simulink model "MotorControl_Bldc"  (R2022a)
settings: Solver=ode4  StartTime=0.0  StopTime=1  FixedStep=Ts/cnt_pTs  RelTol=1e-3
values from neighbouring files (symbols this model uses):
  cnt_pTs = 1000    [motorpara.m]
  Fc = 1/Ts    (= 10000)    [motorpara.m]
  Ki_id = Rs*Fc    (= 4500)    [motorpara.m]
  Ki_iq = Rs*Fc    (= 4500)    [motorpara.m]
  Ki_v = 0.93    [motorpara.m]
  Kp_id = Ls*Fc    (= 4.2)    [motorpara.m]
  Kp_iq = Ls*Fc    (= 4.2)    [motorpara.m]
  Kp_v = 0.05    [motorpara.m]
  Ls = 0.00042    [motorpara.m]
  P = 2    [motorpara.m]
  Rs = 0.45    [motorpara.m]
  SMO_Kslide = 10    [motorpara.m]
  Ts = 1/10000    (= 0.0001)    [motorpara.m]
  V = 12    [motorpara.m]
undefined symbols (not defined in the file or in its folder): DiscIntNeverNeededParam, sigbuilder_block
libraries: nesl_utility x83, fl_lib x67, ee_lib x49, simulink x13, slpidlib x3, mcbplantlib x2, autolibpmsmexterior x1
(part 1 of 4)
settings Model: Creator=gcx  LastModifiedBy=gcx
settings OptimizationCC: DefaultParameterBehavior=Inlined  UseDivisionForNetSlopeComputation=on  GainParamInheritBuiltInType=on  UseFloatMulNetSlope=on  InlineInvariantSignals=on  PassReuseOutputArgsAs=Individual arguments  ZeroExternalMemoryAtStartup=off  ZeroInternalMemoryAtStartup=off  NoFixptDivByZeroProtection=on  EfficientFloat2IntCast=on  LifeSpan=1  OptimizeBlockOrder=speed  DifferentSizesBufferReuse=on  EfficientTunableParamExpr=on
settings DebuggingCC: ParameterTunabilityLossMsg=error
settings HardwareCC: ProdBitPerInt=16  ProdBitPerPointer=16  ProdBitPerSizeT=16  ProdBitPerPtrDiffT=16  ProdLargestAtomicFloat=None  ProdWordSize=16  ProdLongLongMode=on  ProdHWDeviceType=STMicroelectronics->ST10/Super10
settings SFSimCC: MATLABDynamicMemAlloc=off
settings RTWCC: SystemTargetFile=ert.tlc  GenCodeOnly=on  PackageGeneratedCodeAndArtifacts=on  TemplateMakefile=ert_default_tmf
settings CodeAppCC: ForceParamTrailComments=on  IgnoreCustomStorageClasses=off  OperatorAnnotations=on  SimulinkDataObjDesc=on  SFDataObjDesc=on  CustomSymbolStrGlobalVar=rt$N$M  CustomSymbolStrType=$N$M  CustomSymbolStrFcn=$N$M$F  CustomSymbolStrMacro=$N$M  InsertBlockDesc=on
settings ERTTargetCC: TargetLangStandard=C99 (ISO)  GenerateSampleERTMain=on  IncludeMdlTerminateFcn=off  CombineSignalStateStructs=on  CodeInterfacePackaging=Reusable function  SupportComplex=off  SupportNonInlinedSFcns=on  InlinedParameterPlacement=NonHierarchical  ERTCustomFileTemplate=example_file_process.tlc  ERTFilePackagingFormat=CompactWithDataFile

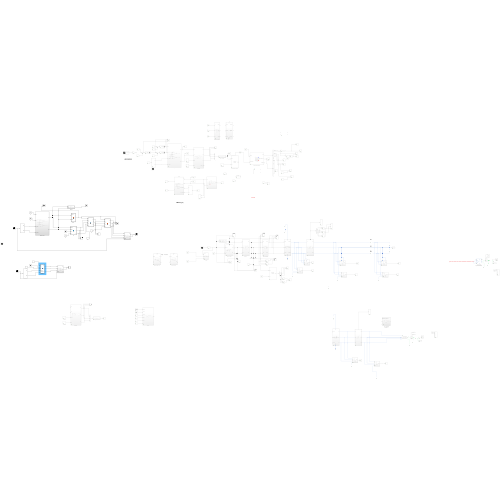
[thumbnail: Simulink's stored preview of the top-level diagram]
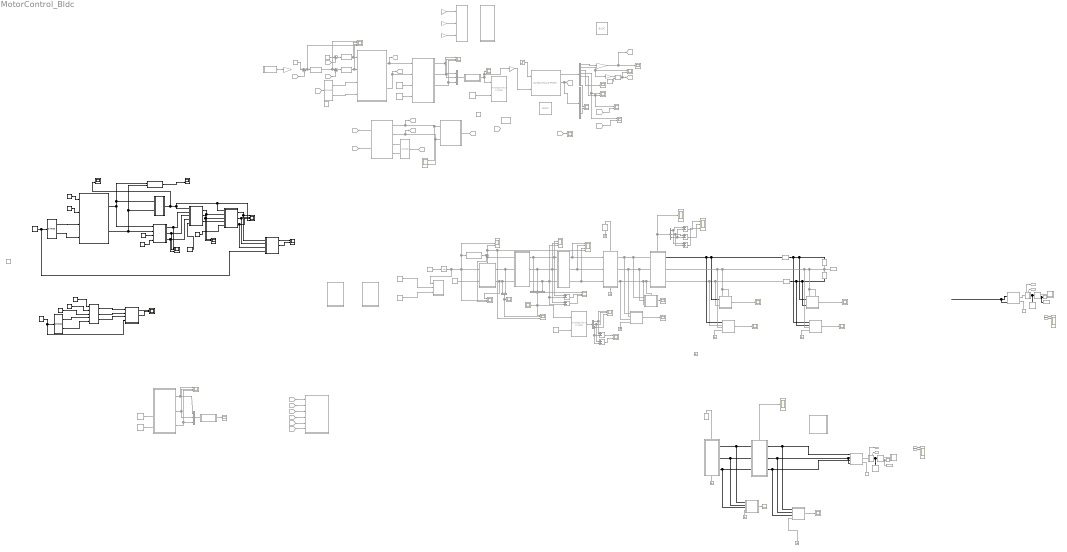
== system MotorControl_Bldc ==
  note: A
  note: 有Bug，可以用来还原
  note: Park变换
  note: 速度测量
  note: ）
  note: C
  note: B
  2Phase_D1D1 : Subsystem  Commented=on
      settings: PortSchema="{\"entries\":[{\"content\":{\"sides\":[{\"content\":{\"connectorIds\":[\"In1\",\"In2\"]},\"type\":\"ConnectorPlacement.EquallySpacedRectSide\",\"uuid\":\"91e4105a-9e8c-434e-97cb-db4fedd585cb\"},{\"content\":{\"connectorIds\":[\"Out1\",\"Out2\"],\"side\":\"RIGHT\"},\"type\":\"ConnectorPlacement.EquallySpacedRectSide\",\"uuid\":\"7c5735c0-a428-475d-8251-3447de6cb9b4\"},{\"content\":{\"connectorIds\":[\"In3\"],\"side\":\"TOP\"},\"type\":\"ConnectorPlacement.EquallySpacedRectSide\",\"uuid\":\"865a6bbc-fe0c-46ed-bd30-e6e1f24b581f\"}]},\"type\":\"ConnectorPlacement.EquallySpacedConnector\",\"uuid\":\"82a7eed4-0b98-4350-8284-359f4eec5efe\"}],\"packageUris\":[\"http://schema.mathworks.com/mf0/Connector/R2020b\"],\"version\":\"1.0\"}"
  2Phase_D1D1_org : Subsystem  Commented=on
      settings: PortSchema="{\"entries\":[{\"content\":{\"sides\":[{\"content\":{\"connectorIds\":[\"In1\",\"In2\"]},\"type\":\"ConnectorPlacement.EquallySpacedRectSide\",\"uuid\":\"91e4105a-9e8c-434e-97cb-db4fedd585cb\"},{\"content\":{\"connectorIds\":[\"Out1\",\"Out2\"],\"side\":\"RIGHT\"},\"type\":\"ConnectorPlacement.EquallySpacedRectSide\",\"uuid\":\"7c5735c0-a428-475d-8251-3447de6cb9b4\"},{\"content\":{\"connectorIds\":[\"In3\"],\"side\":\"TOP\"},\"type\":\"ConnectorPlacement.EquallySpacedRectSide\",\"uuid\":\"865a6bbc-fe0c-46ed-bd30-e6e1f24b581f\"}]},\"type\":\"ConnectorPlacement.EquallySpacedConnector\",\"uuid\":\"82a7eed4-0b98-4350-8284-359f4eec5efe\"}],\"packageUris\":[\"http://schema.mathworks.com/mf0/Connector/R2020b\"],\"version\":\"1.0\"}"
  2Phase_D1D2 : Subsystem  Commented=on
      settings: PortSchema="{\"entries\":[{\"content\":{\"sides\":[{\"content\":{\"connectorIds\":[\"In1\",\"In2\"]},\"type\":\"ConnectorPlacement.EquallySpacedRectSide\",\"uuid\":\"91e4105a-9e8c-434e-97cb-db4fedd585cb\"},{\"content\":{\"connectorIds\":[\"Out1\",\"Out2\"],\"side\":\"RIGHT\"},\"type\":\"ConnectorPlacement.EquallySpacedRectSide\",\"uuid\":\"7c5735c0-a428-475d-8251-3447de6cb9b4\"},{\"content\":{\"connectorIds\":[\"In3\"],\"side\":\"TOP\"},\"type\":\"ConnectorPlacement.EquallySpacedRectSide\",\"uuid\":\"865a6bbc-fe0c-46ed-bd30-e6e1f24b581f\"}]},\"type\":\"ConnectorPlacement.EquallySpacedConnector\",\"uuid\":\"82a7eed4-0b98-4350-8284-359f4eec5efe\"}],\"packageUris\":[\"http://schema.mathworks.com/mf0/Connector/R2020b\"],\"version\":\"1.0\"}"
  2Phase_T : Subsystem  Commented=on
  Add{2..5} (4 alike) : Sum  Commented=on  Inputs=+-
  Add6 : Sum  Commented=on
  Average-Value Inverter : mcbplantlib/Average-Value Inverter  Commented=on
  Average-Value Inverter1 : mcbplantlib/Average-Value Inverter  Commented=on
  BLDC : ee_lib/Electromechanical/Permanent Magnet/BLDC  Commented=on  port_option=ee.enum.threePhasePort.composite  winding_type=ee.enum.statorconnection.delta  rotor_param=ee.enum.pmsm.backemf.trapezoidflux  pm_flux_linkage=0.03 Wb  theta_constant=pi / 12 rad  emf_max=9.6 V  w_meas=600 rpm  DphiDtheta_tab=[0, -.1528, -.1528, .1528, .1528, 0] Wb/rad  back_emf_tab=[0, -9.6, -9.6, 9.6, 9.6, 0] V  rotor_angle_tab=[0, 7.5, 22.5, 37.5, 52.5, 60] deg  nPolePairs=6  axes_param=ee.enum.rotorangle.daxis  stator_param=ee.enum.statorparam.LdLqL0  machine_param=ee.enum.dqparameterization.constant  Ld=0.00022 H  Lq=0.00022 H  idVec=[-200, 0, 200] A  iqVec=[-200, 0, 200] A  LdMatrix=0.00022 * ones(3, 3) H  LqMatrix=0.00022 * ones(3, 3) H  L0=0.00016 H  Ls=0.0002 H  Lm=0 H  Ms=0.00002 H  Rs=0.013 Ohm  zero_sequence=ee.enum.park.zerosequence.include  loss_param=ee.enum.ironloss.none  losses_oc=[0, 0, 0] W  losses_sc=[0, 0, 0] W  f_losses=60 Hz  Isc_losses=95 A  J=0.01 kg*m^2  lam=0 N*m*s/rad  i_d_specify=off  i_d_priority=None  i_d=0 A  i_d_nominal_specify=off  i_d_nominal_unit=A  i_d_nominal_value=1  i_q_specify=off  i_q_priority=None  i_q=0 A  i_q_nominal_specify=off  i_q_nominal_unit=A  i_q_nominal_value=1  torque_specify=off  torque_priority=None  torque=0 N*m  torque_nominal_specify=off  torque_nominal_unit=N*m  torque_nominal_value=1  angular_velocity_specify=off  angular_velocity_priority=High  angular_velocity=0 rpm  angular_velocity_nominal_specify=off  angular_velocity_nominal_unit=rpm  angular_velocity_nominal_value=1  angular_position_specify=off  angular_position_priority=High  angular_position=0 deg  angular_position_nominal_specify=off  angular_position_nominal_unit=deg  angular_position_nominal_value=1  alpha=3.93e-3 1/K  alpha_flux=-0.001 1/K  Tmeas=298.15 K  stator_thermal_mass=100 J/K  rotor_thermal_mass=200 J/K  Rm_percent_rotor=90  Rd_percent_rotor=30  temperatureA_specify=off  temperatureA_priority=High  temperatureA=25 degC  temperatureA_nominal_specify=off  temperatureA_nominal_unit=degC  temperatureA_nominal_value=1  temperatureB_specify=off  temperatureB_priority=High  temperatureB=25 degC  temperatureB_nominal_specify=off  temperatureB_nominal_unit=degC  temperatureB_nominal_value=1  temperatureC_specify=off  temperatureC_priority=High  temperatureC=25 degC  temperatureC_nominal_specify=off  temperatureC_nominal_unit=degC  temperatureC_nominal_value=1  temperatureR_specify=off  temperatureR_priority=High  temperatureR=25 degC  temperatureR_nominal_specify=off  temperatureR_nominal_unit=degC  temperatureR_nominal_value=1
      settings: SourceProductBaseCode=PS  InternalSimscapePortConfiguration="{\"Bottom\":[],\"Left\":[{\"id\":\"N\",\"label\":\"~\",\"type\":\"foundation.electrical.three_phase\"},{\"id\":\"HR\",\"label\":\"HR\",\"type\":\"foundation.thermal.thermal\"}],\"Right\":[{\"id\":\"R\",\"label\":\"R\",\"type\":\"foundation.mechanical.rotational.rotational\"},{\"id\":\"C\",\"label\":\"C\",\"type\":\"foundation.mechanical.rotational.rotational\"},{\"id\":\"HA\",\"label\":\"HA\",\"type\":\"foundation.thermal.thermal\"},{\"id\":\"HB\",\"label\":\"HB\",\"type\":\"foundation.thermal.thermal\"},{\"id\":\"HC\",\"label\":\"HC\",\"type\":\"foundation.thermal.thermal\"}],\"Top\":[]}"
  BLDC1 : ee_lib/Electromechanical/Permanent Magnet/BLDC  Commented=on  port_option=ee.enum.threePhasePort.composite  winding_type=ee.enum.statorconnection.wye  rotor_param=ee.enum.pmsm.backemf.trapezoidflux  pm_flux_linkage=0.03 Wb  theta_constant=pi / 12 rad  emf_max=9.6 V  w_meas=600 rpm  DphiDtheta_tab=[0, -.1528, -.1528, .1528, .1528, 0] Wb/rad  back_emf_tab=[0, -9.6, -9.6, 9.6, 9.6, 0] V  rotor_angle_tab=[0, 7.5, 22.5, 37.5, 52.5, 60] deg  nPolePairs=6  axes_param=ee.enum.rotorangle.daxis  stator_param=ee.enum.statorparam.LdLqL0  machine_param=ee.enum.dqparameterization.constant  Ld=0.00022 H  Lq=0.00022 H  idVec=[-200, 0, 200] A  iqVec=[-200, 0, 200] A  LdMatrix=0.00022 * ones(3, 3) H  LqMatrix=0.00022 * ones(3, 3) H  L0=0.00016 H  Ls=0.0002 H  Lm=0 H  Ms=0.00002 H  Rs=0.013 Ohm  zero_sequence=ee.enum.park.zerosequence.include  loss_param=ee.enum.ironloss.none  losses_oc=[0, 0, 0] W  losses_sc=[0, 0, 0] W  f_losses=60 Hz  Isc_losses=95 A  J=0.01 kg*m^2  lam=0 N*m*s/rad  i_d_specify=off  i_d_priority=None  i_d=0 A  i_d_nominal_specify=off  i_d_nominal_unit=A  i_d_nominal_value=1  i_q_specify=off  i_q_priority=None  i_q=0 A  i_q_nominal_specify=off  i_q_nominal_unit=A  i_q_nominal_value=1  torque_specify=off  torque_priority=None  torque=0 N*m  torque_nominal_specify=off  torque_nominal_unit=N*m  torque_nominal_value=1  angular_velocity_specify=off  angular_velocity_priority=High  angular_velocity=0 rpm  angular_velocity_nominal_specify=off  angular_velocity_nominal_unit=rpm  angular_velocity_nominal_value=1  angular_position_specify=off  angular_position_priority=High  angular_position=0 deg  angular_position_nominal_specify=off  angular_position_nominal_unit=deg  angular_position_nominal_value=1  alpha=3.93e-3 1/K  alpha_flux=-0.001 1/K  Tmeas=298.15 K  stator_thermal_mass=100 J/K  rotor_thermal_mass=200 J/K  Rm_percent_rotor=90  Rd_percent_rotor=30  temperatureA_specify=off  temperatureA_priority=High  temperatureA=25 degC  temperatureA_nominal_specify=off  temperatureA_nominal_unit=degC  temperatureA_nominal_value=1  temperatureB_specify=off  temperatureB_priority=High  temperatureB=25 degC  temperatureB_nominal_specify=off  temperatureB_nominal_unit=degC  temperatureB_nominal_value=1  temperatureC_specify=off  temperatureC_priority=High  temperatureC=25 degC  temperatureC_nominal_specify=off  temperatureC_nominal_unit=degC  temperatureC_nominal_value=1  temperatureR_specify=off  temperatureR_priority=High  temperatureR=25 degC  temperatureR_nominal_specify=off  temperatureR_nominal_unit=degC  temperatureR_nominal_value=1
      settings: SourceProductBaseCode=PS  InternalSimscapePortConfiguration="{\"Bottom\":[],\"Left\":[{\"id\":\"N\",\"label\":\"~\",\"type\":\"foundation.electrical.three_phase\"},{\"id\":\"n\",\"label\":\"n\",\"type\":\"foundation.electrical.electrical\"}],\"Right\":[{\"id\":\"R\",\"label\":\"R\",\"type\":\"foundation.mechanical.rotational.rotational\"},{\"id\":\"C\",\"label\":\"C\",\"type\":\"foundation.mechanical.rotational.rotational\"}],\"Top\":[]}"
  Bus Selector : BusSelector  Commented=on  OutputSignals=MtrSpd,MtrPos,MtrTrq,IdSync,IqSync,IaStator,IbStator,IcStator
  Constant : Constant  Value=10
  Constant1 : Constant  Commented=on  Value=2000
  Constant10 : Constant  Commented=on  Value=V
  Constant11 : Constant  Value=3
  Constant2 : Constant  Commented=on  Value=Ts  VectorParams1D=off  SampleTime=-1
  Constant3 : Constant  Commented=on  Value=V  VectorParams1D=off  SampleTime=-1
  Constant4 : Constant  Commented=on  Value=V  VectorParams1D=off  SampleTime=-1
  Constant5 : Constant  Value=4
  Constant6 : Constant  Commented=on  Value=2*pi
  Constant7 : Constant  Commented=on  Value=0
  Constant8 : Constant  Commented=on  Value=V  VectorParams1D=off  SampleTime=-1
  Constant9 : Constant  Commented=on  VectorParams1D=off  SampleTime=-1
  Crrent : Goto  Commented=on  GotoTag=PhI
  D : Constant  Value=4
  DC Voltage Source : ee_lib/Additional Components/SPICE Sources/DC Voltage Source  Commented=on  DC=380 V
  DC Voltage Source1 : ee_lib/Additional Components/SPICE Sources/DC Voltage Source  Commented=on  DC=380 V
  Da-Dc : Sum  Commented=on  Inputs=+-
  Db-Dc : Sum  Commented=on  Inputs=+-
  Demux : Demux  Commented=on  Outputs=3
  Demux1 : Demux  Commented=on  Outputs=3
  Demux2 : Demux  Commented=on  Outputs=3
  Duty_conver : Subsystem  Commented=on
  Duty_conver1 : Subsystem  Commented=on
  Electrical Reference{,1..8} (9 alike) : fl_lib/Electrical/Electrical Elements/Electrical Reference  Commented=on
      settings: SourceProductBaseCode=PW,SS,VE
  From1 : From  Commented=on  GotoTag=PhI
  From10 : From  Commented=on  GotoTag=Theta
  From11 : From  Commented=on  GotoTag=V
  From12 : From  Commented=on  GotoTag=V
  From13 : From  Commented=on  GotoTag=Id
  From14 : From  Commented=on  GotoTag=Tq
  From15 : From  Commented=on  GotoTag=Iq
  From16 : From  Commented=on  GotoTag=w
  From17 : From  Commented=on  GotoTag=Tq
  From18 : From  Commented=on  GotoTag=w
  From19 : From  Commented=on  GotoTag=PhI
  From2 : From  Commented=on  GotoTag=Theta
  From20 : From  Commented=on  GotoTag=Theta
  From3 : From  Commented=on  GotoTag=Id
  From4 : From  Commented=on  GotoTag=Iq
  From5 : From  Commented=on  GotoTag=V
  From6 : From  Commented=on  GotoTag=Valpha
  From7 : From  Commented=on  GotoTag=Vbeta
  From8 : From  Commented=on  GotoTag=Ialpha
  From9 : From  Commented=on  GotoTag=Ibeta
  Function Caller : FunctionCaller  Commented=on  FunctionPrototype=y = f(u)  InputArgumentSpecifications=<Enter example>  OutputArgumentSpecifications=<Enter example>
  Gain : Gain  Commented=on  Gain=2/pi*60/P
  Gain1 : Gain  Commented=on  Gain=P
  Gain2 : Gain  Commented=on  Gain=24
  Gain3 : Gain  Commented=on  Gain=2000
  Gain4 : Gain  Commented=on  Gain=1/Ts
  Gain5 : Gain  Commented=on  Gain=1/Ts
  Gain6 : Gain  Commented=on  Gain=1/Ts
  Goto : Goto  Commented=on  GotoTag=Id
  Goto1 : Goto  Commented=on  GotoTag=Iq
  Goto10 : Goto  Commented=on  GotoTag=Tq
  Goto2 : Goto  Commented=on  GotoTag=V
  Goto3 : Goto  Commented=on  GotoTag=Valpha
  Goto4 : Goto  Commented=on  GotoTag=Vbeta
  Goto5 : Goto  Commented=on  GotoTag=Ialpha
  Goto6 : Goto  Commented=on  GotoTag=Ibeta
  Goto7 : Goto  Commented=on  GotoTag=Tq
  Goto8 : Goto  Commented=on  GotoTag=w
  Goto9 : Goto  Commented=on  GotoTag=w
  Inductor3 : ee_lib/Passive/Inductor  Commented=on  l=1e-3 H  enable_L_tol=0  L_tol=20  tol_distribution=1  nSigma=4  r=0 Ohm  g=1e-9 1/Ohm  enable_operating_limits=0  operating_limit_action=2  max_working_current=1 A  power_rating=1 W  enable_faults=0  fault_action=1  lambdaPercent=50  k_faulted=0.9999  turnsShort=0  openCct=0  groundShort=0  groundShortG=0 1/Ohm  tau_fault=1e-3 s  enable_temporal_fault=0  t_fault=1 s  enable_behavioral_fault=0  max_permissible_voltage=100 V  n_fail_on_voltage=1  max_permissible_current=1 A  t_fail_on_current=1 s  i_L_specify=off  i_L_priority=High  i_L=0 A  i_L_nominal_specify=off  i_L_nominal_unit=A  i_L_nominal_value=1
  Inductor4 : ee_lib/Passive/Inductor  Commented=on  l=1e-3 H  enable_L_tol=0  L_tol=20  tol_distribution=1  nSigma=4  r=0 Ohm  g=1e-9 1/Ohm  enable_operating_limits=0  operating_limit_action=2  max_working_current=1 A  power_rating=1 W  enable_faults=0  fault_action=1  lambdaPercent=50  k_faulted=0.9999  turnsShort=0  openCct=0  groundShort=0  groundShortG=0 1/Ohm  tau_fault=1e-3 s  enable_temporal_fault=0  t_fault=1 s  enable_behavioral_fault=0  max_permissible_voltage=100 V  n_fail_on_voltage=1  max_permissible_current=1 A  t_fail_on_current=1 s  i_L_specify=off  i_L_priority=High  i_L=0 A  i_L_nominal_specify=off  i_L_nominal_unit=A  i_L_nominal_value=1
  Inertia1 : fl_lib/Mechanical/Rotational Elements/Inertia  Commented=on  inertia=0.0146 kg*m^2  num_ports=foundation.enum.numPorts2.one  w_specify=on  w_priority=High  w=0 rpm  w_nominal_specify=off  w_nominal_unit=rad/s  w_nominal_value=1  t_specify=off  t_priority=High  t=0 N*m  t_nominal_specify=off  t_nominal_unit=N*m  t_nominal_value=1
      settings: SourceProductBaseCode=PW,SS,VE
  Inertia3 : fl_lib/Mechanical/Rotational Elements/Inertia  Commented=on  inertia=0.0146 kg*m^2  num_ports=foundation.enum.numPorts2.one  w_specify=on  w_priority=High  w=0 rpm  w_nominal_specify=off  w_nominal_unit=rad/s  w_nominal_value=1  t_specify=off  t_priority=High  t=0 N*m  t_nominal_specify=off  t_nominal_unit=N*m  t_nominal_value=1
      settings: SourceProductBaseCode=PW,SS,VE
  Inverse_Park : Subsystem  Commented=on
  Inverse_Park1 : Subsystem
  MRRef IPMSM1 : fl_lib/Mechanical/Rotational Elements/Mechanical Rotational Reference  Commented=on
      settings: SourceProductBaseCode=PW,SS,VE
  MRRef IPMSM3 : fl_lib/Mechanical/Rotational Elements/Mechanical Rotational Reference  Commented=on
      settings: SourceProductBaseCode=PW,SS,VE
  MRRef Load1 : fl_lib/Mechanical/Rotational Elements/Mechanical Rotational Reference  Commented=on
      settings: SourceProductBaseCode=PW,SS,VE
  MRRef Load3 : fl_lib/Mechanical/Rotational Elements/Mechanical Rotational Reference  Commented=on
      settings: SourceProductBaseCode=PW,SS,VE
  Math Function : Math  Commented=on
  Mod : Math  Commented=on  Operator=mod
  Mux : Mux  Commented=on  Inputs=3
  Mux1 : Mux  Commented=on  Inputs=3
  Mux2 : Mux  Commented=on  Inputs=3
  Mux3 : Mux  Commented=on  Inputs=2
  PID Controller : slpidlib/PID Controller  Commented=on  Controller=PID  Form=Parallel  TimeDomain=Discrete-time  UseExternalTs=off  SampleTime=1/Fc  IntegratorMethod=Forward Euler  FilterMethod=Forward Euler  ControllerParametersSource=internal  P=Kp_id  I=Ki_id  UseKiTs=off  D=0  N=100  UseFilter=on  TunerSelectOption=Transfer Function Based (PID Tuner App)  InitialConditionSource=internal  InitialConditionForIntegrator=0  InitialConditionForFilter=0  DifferentiatorICPrevScaledInput=0  ExternalReset=none  TrackingMode=off  Kt=1  LimitOutput=on  SatLimitsSource=internal  UpperSaturationLimit=V/sqrt(3)  LowerSaturationLimit=-V/sqrt(3)  LinearizeAsGain=on  AntiWindupMode=none  Kb=1  POutMin=[]  POutMax=[]  IOutMin=[]  IOutMax=[]  DOutMin=[]  DOutMax=[]  NOutMin=[]  NOutMax=[]  SumOutMin=[]  SumOutMax=[]  SaturationOutMin=[]  SaturationOutMax=[]  PParamMin=[]  PParamMax=[]  IParamMin=[]  IParamMax=[]  DParamMin=[]  DParamMax=[]  NParamMin=[]  NParamMax=[]  KbParamMin=[]  KbParamMax=[]  KtParamMin=[]  KtParamMax=[]  KbOutMin=[]  KbOutMax=[]  KtOutMin=[]  KtOutMax=[]  IntegratorOutMin=[]  IntegratorOutMax=[]  FilterOutMin=[]  FilterOutMax=[]  SumI1OutMin=[]  SumI1OutMax=[]  SumI2OutMin=[]  SumI2OutMax=[]  SumI3OutMin=[]  SumI3OutMax=[]  SumI4OutMin=[]  SumI4OutMax=[]  SumDOutMin=[]  SumDOutMax=[]  DifferentiatorOutMin=[]  DifferentiatorOutMax=[]  FilterDiffOutCoefMin=[]  FilterDiffOutCoefMax=[]  ReciprocalOutMin=[]  ReciprocalOutMax=[]  SumDenOutMin=[]  SumDenOutMax=[]  SumNumOutMin=[]  SumNumOutMax=[]  DivideOutMin=[]  DivideOutMax=[]  UdiffTsProdOutMin=[]  UdiffTsProdOutMax=[]  NTsProdOutMin=[]  NTsProdOutMax=[]  UintegralTsProdOutMin=[]  UintegralTsProdOutMax=[]  UngainTsProdOutMin=[]  UngainTsProdOutMax=[]  IntegratorContinuousStateAttributes=''  IntegratorStateMustResolveToSignalObject=off  IntegratorRTWStateStorageClass=Auto  FilterContinuousStateAttributes=''  FilterStateMustResolveToSignalObject=off  FilterRTWStateStorageClass=Auto  ParallelPVariant=InternalParameters  IdealPVariant=Disabled  IVariant=InternalParameters  DVariant=InternalParameters  IntegratorVariant=Discrete  SatVariant=Enabled  AWVariant=Passthrough  PCopyVariant=Disabled  TRVariant=Disabled  FdbkBlocksVariant=Forward  IdealPFdbkVariant=Disabled  SatFdbkVariant=Disabled  DerivativeFilterVariant=ForwardEulerFilter  NVariant=InternalParameters  NCopyVariant=Disabled  FilterICVariant=InternalICsFilter  IntegratorICVariant=InternalICs  ExternalResetVariant=Disabled  TRSumVariant=Passthrough  SumFdbkVariant=Disabled  SumVariant=Sum_PID  TsampFilterVariant=InternalTs  TsampNgainVariant=Passthrough  TsampIntegralVariant=Passthrough  ExternalSaturationOutDataTypeStr=Inherit: Same as second input  aMode=0
  PID Controller1 : slpidlib/PID Controller  Commented=on  Controller=PID  Form=Parallel  TimeDomain=Discrete-time  UseExternalTs=off  SampleTime=1/Fc  IntegratorMethod=Forward Euler  FilterMethod=Forward Euler  ControllerParametersSource=internal  P=Kp_v  I=Ki_v  UseKiTs=off  D=0  N=100  UseFilter=on  TunerSelectOption=Transfer Function Based (PID Tuner App)  InitialConditionSource=internal  InitialConditionForIntegrator=0  InitialConditionForFilter=0  DifferentiatorICPrevScaledInput=0  ExternalReset=none  TrackingMode=off  Kt=1  LimitOutput=on  SatLimitsSource=internal  UpperSaturationLimit=20  LowerSaturationLimit=-20  LinearizeAsGain=on  AntiWindupMode=none  Kb=1  POutMin=[]  POutMax=[]  IOutMin=[]  IOutMax=[]  DOutMin=[]  DOutMax=[]  NOutMin=[]  NOutMax=[]  SumOutMin=[]  SumOutMax=[]  SaturationOutMin=[]  SaturationOutMax=[]  PParamMin=[]  PParamMax=[]  IParamMin=[]  IParamMax=[]  DParamMin=[]  DParamMax=[]  NParamMin=[]  NParamMax=[]  KbParamMin=[]  KbParamMax=[]  KtParamMin=[]  KtParamMax=[]  KbOutMin=[]  KbOutMax=[]  KtOutMin=[]  KtOutMax=[]  IntegratorOutMin=[]  IntegratorOutMax=[]  FilterOutMin=[]  FilterOutMax=[]  SumI1OutMin=[]  SumI1OutMax=[]  SumI2OutMin=[]  SumI2OutMax=[]  SumI3OutMin=[]  SumI3OutMax=[]  SumI4OutMin=[]  SumI4OutMax=[]  SumDOutMin=[]  SumDOutMax=[]  DifferentiatorOutMin=[]  DifferentiatorOutMax=[]  FilterDiffOutCoefMin=[]  FilterDiffOutCoefMax=[]  ReciprocalOutMin=[]  ReciprocalOutMax=[]  SumDenOutMin=[]  SumDenOutMax=[]  SumNumOutMin=[]  SumNumOutMax=[]  DivideOutMin=[]  DivideOutMax=[]  UdiffTsProdOutMin=[]  UdiffTsProdOutMax=[]  NTsProdOutMin=[]  NTsProdOutMax=[]  UintegralTsProdOutMin=[]  UintegralTsProdOutMax=[]  UngainTsProdOutMin=[]  UngainTsProdOutMax=[]  IntegratorContinuousStateAttributes=''  IntegratorStateMustResolveToSignalObject=off  IntegratorRTWStateStorageClass=Auto  FilterContinuousStateAttributes=''  FilterStateMustResolveToSignalObject=off  FilterRTWStateStorageClass=Auto  ParallelPVariant=InternalParameters  IdealPVariant=Disabled  IVariant=InternalParameters  DVariant=InternalParameters  IntegratorVariant=Discrete  SatVariant=Enabled  AWVariant=Passthrough  PCopyVariant=Disabled  TRVariant=Disabled  FdbkBlocksVariant=Forward  IdealPFdbkVariant=Disabled  SatFdbkVariant=Disabled  DerivativeFilterVariant=ForwardEulerFilter  NVariant=InternalParameters  NCopyVariant=Disabled  FilterICVariant=InternalICsFilter  IntegratorICVariant=InternalICs  ExternalResetVariant=Disabled  TRSumVariant=Passthrough  SumFdbkVariant=Disabled  SumVariant=Sum_PID  TsampFilterVariant=InternalTs  TsampNgainVariant=Passthrough  TsampIntegralVariant=Passthrough  ExternalSaturationOutDataTypeStr=Inherit: Same as second input  aMode=0
  PID Controller2 : slpidlib/PID Controller  Commented=on  Controller=PID  Form=Parallel  TimeDomain=Discrete-time  UseExternalTs=off  SampleTime=1/Fc  IntegratorMethod=Forward Euler  FilterMethod=Forward Euler  ControllerParametersSource=internal  P=Kp_iq  I=Ki_iq  UseKiTs=off  D=0  N=100  UseFilter=on  TunerSelectOption=Transfer Function Based (PID Tuner App)  InitialConditionSource=internal  InitialConditionForIntegrator=0  InitialConditionForFilter=0  DifferentiatorICPrevScaledInput=0  ExternalReset=none  TrackingMode=off  Kt=1  LimitOutput=on  SatLimitsSource=internal  UpperSaturationLimit=V/sqrt(3)  LowerSaturationLimit=-V/sqrt(3)  LinearizeAsGain=on  AntiWindupMode=none  Kb=1  POutMin=[]  POutMax=[]  IOutMin=[]  IOutMax=[]  DOutMin=[]  DOutMax=[]  NOutMin=[]  NOutMax=[]  SumOutMin=[]  SumOutMax=[]  SaturationOutMin=[]  SaturationOutMax=[]  PParamMin=[]  PParamMax=[]  IParamMin=[]  IParamMax=[]  DParamMin=[]  DParamMax=[]  NParamMin=[]  NParamMax=[]  KbParamMin=[]  KbParamMax=[]  KtParamMin=[]  KtParamMax=[]  KbOutMin=[]  KbOutMax=[]  KtOutMin=[]  KtOutMax=[]  IntegratorOutMin=[]  IntegratorOutMax=[]  FilterOutMin=[]  FilterOutMax=[]  SumI1OutMin=[]  SumI1OutMax=[]  SumI2OutMin=[]  SumI2OutMax=[]  SumI3OutMin=[]  SumI3OutMax=[]  SumI4OutMin=[]  SumI4OutMax=[]  SumDOutMin=[]  SumDOutMax=[]  DifferentiatorOutMin=[]  DifferentiatorOutMax=[]  FilterDiffOutCoefMin=[]  FilterDiffOutCoefMax=[]  ReciprocalOutMin=[]  ReciprocalOutMax=[]  SumDenOutMin=[]  SumDenOutMax=[]  SumNumOutMin=[]  SumNumOutMax=[]  DivideOutMin=[]  DivideOutMax=[]  UdiffTsProdOutMin=[]  UdiffTsProdOutMax=[]  NTsProdOutMin=[]  NTsProdOutMax=[]  UintegralTsProdOutMin=[]  UintegralTsProdOutMax=[]  UngainTsProdOutMin=[]  UngainTsProdOutMax=[]  IntegratorContinuousStateAttributes=''  IntegratorStateMustResolveToSignalObject=off  IntegratorRTWStateStorageClass=Auto  FilterContinuousStateAttributes=''  FilterStateMustResolveToSignalObject=off  FilterRTWStateStorageClass=Auto  ParallelPVariant=InternalParameters  IdealPVariant=Disabled  IVariant=InternalParameters  DVariant=InternalParameters  IntegratorVariant=Discrete  SatVariant=Enabled  AWVariant=Passthrough  PCopyVariant=Disabled  TRVariant=Disabled  FdbkBlocksVariant=Forward  IdealPFdbkVariant=Disabled  SatFdbkVariant=Disabled  DerivativeFilterVariant=ForwardEulerFilter  NVariant=InternalParameters  NCopyVariant=Disabled  FilterICVariant=InternalICsFilter  IntegratorICVariant=InternalICs  ExternalResetVariant=Disabled  TRSumVariant=Passthrough  SumFdbkVariant=Disabled  SumVariant=Sum_PID  TsampFilterVariant=InternalTs  TsampNgainVariant=Passthrough  TsampIntegralVariant=Passthrough  ExternalSaturationOutDataTypeStr=Inherit: Same as second input  aMode=0
  PWM_Generator : Subsystem  Commented=on
  PWM_Generator1 : Subsystem  Commented=on
  Park : Subsystem  Commented=on
  Q : Constant  Value=3
  Q1 : Constant  Value=10
  Q2 : Constant
  Q3 : Constant
  Q4 : Constant
  Repeating Sequence : simulink/Sources/Repeating Sequence  Commented=on  rep_seq_t=[0 1]  rep_seq_y=[0 2*pi()]
  Repeating Sequence1 : simulink/Sources/Repeating Sequence  Commented=on  rep_seq_t=[0 0.01]  rep_seq_y=[2*pi 0]
  Repeating Sequence2 : simulink/Sources/Repeating Sequence  Commented=on  rep_seq_t=[0 1]  rep_seq_y=[0 2*pi()]
  Repeating Sequence3 : simulink/Sources/Repeating Sequence  rep_seq_t=[0 0.1]  rep_seq_y=[0 2*pi()]
  Repeating Sequence4 : simulink/Sources/Repeating Sequence  rep_seq_t=[0 0.1]  rep_seq_y=[0 2*pi()]
  Resistor2 : ee_lib/Passive/Resistor  Commented=on  R=1 Ohm  enable_R_tol=0  R_tol=5  tol_distribution=1  nSigma=4  enable_operating_limits=0  operating_limit_action=2  max_working_voltage=100 V  power_rating=1 W  enable_faults=0  fault_action=1  R_faulted=inf Ohm  enable_temporal_fault=0  t_fault=1 s  enable_behavioral_fault=0  max_permissible_current=1 A  t_fail_on_current=1 s  noise_mode=0  sample_time=1e-3 s  repeatability=1  auto_seed=2715962282  user_seed=0  Tdevice=25 degC  power_derating_T1=70 degC  power_derating_T2=155 degC  operating_temperature_range_vec=[-50, 150] degC  alpha=3.93e-3 1/K  Tmeas=25 degC  thermal_mass=100 J/K  temperature_specify=off  temperature_priority=High  temperature=298.15 K  temperature_nominal_specify=off  temperature_nominal_unit=K  temperature_nominal_value=1
  Resistor3 : ee_lib/Passive/Resistor  Commented=on  R=1 Ohm  enable_R_tol=0  R_tol=5  tol_distribution=1  nSigma=4  enable_operating_limits=0  operating_limit_action=2  max_working_voltage=100 V  power_rating=1 W  enable_faults=0  fault_action=1  R_faulted=inf Ohm  enable_temporal_fault=0  t_fault=1 s  enable_behavioral_fault=0  max_permissible_current=1 A  t_fail_on_current=1 s  noise_mode=0  sample_time=1e-3 s  repeatability=1  auto_seed=418932850  user_seed=0  Tdevice=25 degC  power_derating_T1=70 degC  power_derating_T2=155 degC  operating_temperature_range_vec=[-50, 150] degC  alpha=3.93e-3 1/K  Tmeas=25 degC  thermal_mass=100 J/K  temperature_specify=off  temperature_priority=High  temperature=298.15 K  temperature_nominal_specify=off  temperature_nominal_unit=K  temperature_nominal_value=1
  SMO : Subsystem  Commented=on
  SVPWM : Subsystem  Commented=on
  SVPWM1 : Subsystem  Commented=on
  Scope{,1..2,7,10..11,31,36} (8 alike) : Scope  Commented=on  NumInputPorts=2
  Scope12 : Scope  Commented=on  NumInputPorts=4
  Scope{3..4,13..14,16,19,21,29} (8 alike) : Scope  Commented=on  NumInputPorts=3
  Scope{5..6,8..9,15,18,20,22..23,25..27,30,32..34} (16 alike) : Scope  Commented=on
  Scope17 : Scope  Commented=on  NumInputPorts=4
  Scope24 : Scope  Commented=on  NumInputPorts=6
  Scope28 : Scope  Commented=on  NumInputPorts=4
  Scope35 : Scope  Commented=on  NumInputPorts=6
  Scope37 : Scope  NumInputPorts=4
  Scope{38,40..41,44} (4 alike) : Scope  NumInputPorts=3
  Scope39 : Scope  NumInputPorts=4
  Scope45 : Scope  NumInputPorts=4
  Sector : MATLAB Function  TreatAsAtomicUnit=on
  Sector1 : Subsystem  Commented=on
  Sector2 : Subsystem
  Sector3 : MATLAB Function  TreatAsAtomicUnit=on
  Sensing trq1 : Subsystem  Commented=on
      settings: PortSchema="{\"entries\":[{\"content\":{\"sides\":[{\"content\":{\"connectorIds\":[\"LConn1\"]},\"type\":\"ConnectorPlacement.EquallySpacedRectSide\",\"uuid\":\"c5057f2e-2c18-4118-b873-a75143a124e4\"},{\"content\":{\"connectorIds\":[\"RConn1\"],\"side\":\"RIGHT\"},\"type\":\"ConnectorPlacement.EquallySpacedRectSide\",\"uuid\":\"847dbac9-66f5-462a-b095-b42c8738b9ce\"},{\"content\":{\"connectorIds\":[\"Out1\",\"Out2\"],\"side\":\"TOP\"},\"type\":\"ConnectorPlacement.EquallySpacedRectSide\",\"uuid\":\"1cd52aa7-c39c-45ef-b799-a348546c5bc9\"}]},\"type\":\"ConnectorPlacement.EquallySpacedConnector\",\"uuid\":\"7d89bf63-b784-4419-8d3e-10ce7abb2518\"}],\"packageUris\":[\"http://schema.mathworks.com/mf0/Connector/R2020b\"],\"version\":\"1.0\"}"
  Sensing trq3 : Subsystem  Commented=on
      settings: PortSchema="{\"entries\":[{\"content\":{\"sides\":[{\"content\":{\"connectorIds\":[\"LConn1\"]},\"type\":\"ConnectorPlacement.EquallySpacedRectSide\",\"uuid\":\"c5057f2e-2c18-4118-b873-a75143a124e4\"},{\"content\":{\"connectorIds\":[\"RConn1\"],\"side\":\"RIGHT\"},\"type\":\"ConnectorPlacement.EquallySpacedRectSide\",\"uuid\":\"847dbac9-66f5-462a-b095-b42c8738b9ce\"},{\"content\":{\"connectorIds\":[\"Out1\",\"Out2\"],\"side\":\"TOP\"},\"type\":\"ConnectorPlacement.EquallySpacedRectSide\",\"uuid\":\"1cd52aa7-c39c-45ef-b799-a348546c5bc9\"}]},\"type\":\"ConnectorPlacement.EquallySpacedConnector\",\"uuid\":\"7d89bf63-b784-4419-8d3e-10ce7abb2518\"}],\"packageUris\":[\"http://schema.mathworks.com/mf0/Connector/R2020b\"],\"version\":\"1.0\"}"
  Signal Builder : Subsystem  Tag=STV Subsys  Commented=on  LoadFcn=sigbuilder_block('load');  StartFcn=sigbuilder_block('start');  StopFcn=sigbuilder_block('stop');  ClipboardFcn=sigbuilder_block('clipboard');  mask(Sigbuilder block){tuvar=[0:10]}
      mask help: Simulink:masks:SigbuilderBlock_MD
      mask init:
      | if ~strcmp(get_param(bdroot(gcbh),'SimulationStatus'),'stopped') tuvar = sigbuilder_block('maskInit'); end
      settings: CopyFcn=sigbuilder_block('copy');  DeleteFcn=sigbuilder_block('delete');  ModelCloseFcn=sigbuilder_block('modelClose');  PreSaveFcn=sigbuilder_block('preSave');  PauseFcn=sigbuilder_block('pause');  ContinueFcn=sigbuilder_block('continue');  NameChangeFcn=sigbuilder_block('namechange');  OpenFcn=sigbuilder_block('open',[391.2 110.4 550.8 400.2 ]);  CloseFcn=sigbuilder_block('close');
      mask Display: plot(0, 0, 100, 100,[2, 2, 32, 32, 2], [68, 8, 8, 68, 68],[32, 2], [38, 38], [32, 19, 2],[53, 60, 44], [32, 17, 17, 2],[16, 16, 31, 31]);txt = getActiveGroup(gcbh);text(2, 100, txt,'verticalAlignment', 'top');
  SinCos : Trigonometry  Operator=sincos
  SinCos1 : Trigonometry  Commented=on  Operator=sincos
  SinCos2 : Trigonometry  Commented=on  Operator=sincos
  SinCos3 : Trigonometry  Operator=sincos
  "Single-Phase Asynchronous Machine (fundamental, SI)1" : ee_lib/Electromechanical/Asynchronous/Induction Machine (Single-Phase)  Commented=on  type_option=ee.enum.asm.singlePhaseConfig.twowindings  SRated=SRated V*A  VRated=VRated V  FRated=FRated Hz  nPolePairs=p  param_unit=ee.enum.unit.si  Ras=Ras Ohm  Llas=Llas H  Rar=Rar Ohm  Llar=Llar uH  Lms=Lms uH  Rbs=Rbs Ohm  Llbs=Llbs uH  pu_Ras=0.0135  pu_Llas=0.0188  pu_Rar=0.0276  pu_Llar=0.0140  pu_Lms=0.4472  pu_Rbs=0.0478  pu_Llbs=0.0216  a=a  Rs=3 Ohm  Cs=0.00018 F  Rr=9 Ohm  Cr=0.000015 F  pu_Rs=0.0223  pu_Cs=9.1232  pu_Rr=0.0669  pu_Cr=0.7603  wd=80  J=0 kg*m^2  lam=0 N*m/(rad/s)  angular_position_specify=off  angular_position_priority=None  angular_position=0 deg  angular_position_nominal_specify=off  angular_position_nominal_unit=deg  angular_position_nominal_value=1  psids_specify=off  psids_priority=None  psids=0 Wb  psids_nominal_specify=off  psids_nominal_unit=Wb  psids_nominal_value=1  psiqs_specify=off  psiqs_priority=None  psiqs=0 Wb  psiqs_nominal_specify=off  psiqs_nominal_unit=Wb  psiqs_nominal_value=1  psidr_specify=off  psidr_priority=None  psidr=0 Wb  psidr_nominal_specify=off  psidr_nominal_unit=Wb  psidr_nominal_value=1  psiqr_specify=off  psiqr_priority=None  psiqr=0 Wb  psiqr_nominal_specify=off  psiqr_nominal_unit=Wb  psiqr_nominal_value=1  pu_psiqs_specify=off  pu_psiqs_priority=None  pu_psiqs=0  pu_psiqs_nominal_specify=off  pu_psiqs_nominal_unit=1  pu_psiqs_nominal_value=1  pu_psids_specify=off  pu_psids_priority=None  pu_psids=0  pu_psids_nominal_specify=off  pu_psids_nominal_unit=1  pu_psids_nominal_value=1  pu_psiqr_specify=off  pu_psiqr_priority=None  pu_psiqr=0  pu_psiqr_nominal_specify=off  pu_psiqr_nominal_unit=1  pu_psiqr_nominal_value=1  pu_psidr_specify=off  pu_psidr_priority=None  pu_psidr=0  pu_psidr_nominal_specify=off  pu_psidr_nominal_unit=1  pu_psidr_nominal_value=1  Tmeas=298.15 K  alpha=3.93e-3 1/K  alpha_cage=4.4e-3 1/K  stator_thermal_mass=100 J/K  rotor_thermal_mass=200 J/K  temperatureA_specify=off  temperatureA_priority=High  temperatureA=25 degC  temperatureA_nominal_specify=off  temperatureA_nominal_unit=degC  temperatureA_nominal_value=1  temperatureB_specify=off  temperatureB_priority=High  temperatureB=25 degC  temperatureB_nominal_specify=off  temperatureB_nominal_unit=degC  temperatureB_nominal_value=1  temperatureR_specify=off  temperatureR_priority=High  temperatureR=25 degC  temperatureR_nominal_specify=off  temperatureR_nominal_unit=degC  temperatureR_nominal_value=1
      settings: SourceProductBaseCode=PS  InternalSimscapePortConfiguration="{\"Bottom\":[],\"Left\":[{\"id\":\"a1\",\"label\":\"a1\",\"type\":\"foundation.electrical.electrical\"},{\"id\":\"a2\",\"label\":\"a2\",\"type\":\"foundation.electrical.electrical\"},{\"id\":\"b1\",\"label\":\"b1\",\"type\":\"foundation.electrical.electrical\"},{\"id\":\"b2\",\"label\":\"b2\",\"type\":\"foundation.electrical.electrical\"}],\"Right\":[{\"id\":\"pu_output\",\"label\":\"pu\",\"type\":\"output\"},{\"id\":\"R\",\"label\":\"R\",\"type\":\"foundation.mechanical.rotational.rotational\"},{\"id\":\"C\",\"label\":\"C\",\"type\":\"foundation.mechanical.rotational.rotational\"}],\"Top\":[]}"
  "Single-Phase Asynchronous Machine (fundamental, SI)4" : ee_lib/Electromechanical/Asynchronous/Induction Machine (Single-Phase)  Commented=on  type_option=ee.enum.asm.singlePhaseConfig.twowindings  SRated=1000 V*A  VRated=220 V  FRated=50 Hz  nPolePairs=4  param_unit=ee.enum.unit.si  Ras=1 Ohm  Llas=0.01 H  Rar=0.1 Ohm  Llar=1 uH  Lms=0.01 H  Rbs=0.1 Ohm  Llbs=1 uH  pu_Ras=0.0135  pu_Llas=0.0188  pu_Rar=0.0276  pu_Llar=0.0140  pu_Lms=0.4472  pu_Rbs=0.0478  pu_Llbs=0.0216  a=1  Rs=3 Ohm  Cs=0.00018 F  Rr=9 Ohm  Cr=0.000015 F  pu_Rs=0.0223  pu_Cs=9.1232  pu_Rr=0.0669  pu_Cr=0.7603  wd=80  J=0 kg*m^2  lam=0 N*m/(rad/s)  angular_position_specify=off  angular_position_priority=None  angular_position=0 deg  angular_position_nominal_specify=off  angular_position_nominal_unit=deg  angular_position_nominal_value=1  psids_specify=off  psids_priority=None  psids=0 Wb  psids_nominal_specify=off  psids_nominal_unit=Wb  psids_nominal_value=1  psiqs_specify=off  psiqs_priority=None  psiqs=0 Wb  psiqs_nominal_specify=off  psiqs_nominal_unit=Wb  psiqs_nominal_value=1  psidr_specify=off  psidr_priority=None  psidr=0 Wb  psidr_nominal_specify=off  psidr_nominal_unit=Wb  psidr_nominal_value=1  psiqr_specify=off  psiqr_priority=None  psiqr=0 Wb  psiqr_nominal_specify=off  psiqr_nominal_unit=Wb  psiqr_nominal_value=1  pu_psiqs_specify=off  pu_psiqs_priority=None  pu_psiqs=0  pu_psiqs_nominal_specify=off  pu_psiqs_nominal_unit=1  pu_psiqs_nominal_value=1  pu_psids_specify=off  pu_psids_priority=None  pu_psids=0  pu_psids_nominal_specify=off  pu_psids_nominal_unit=1  pu_psids_nominal_value=1  pu_psiqr_specify=off  pu_psiqr_priority=None  pu_psiqr=0  pu_psiqr_nominal_specify=off  pu_psiqr_nominal_unit=1  pu_psiqr_nominal_value=1  pu_psidr_specify=off  pu_psidr_priority=None  pu_psidr=0  pu_psidr_nominal_specify=off  pu_psidr_nominal_unit=1  pu_psidr_nominal_value=1  Tmeas=298.15 K  alpha=3.93e-3 1/K  alpha_cage=4.4e-3 1/K  stator_thermal_mass=100 J/K  rotor_thermal_mass=200 J/K  temperatureA_specify=off  temperatureA_priority=High  temperatureA=25 degC  temperatureA_nominal_specify=off  temperatureA_nominal_unit=degC  temperatureA_nominal_value=1  temperatureB_specify=off  temperatureB_priority=High  temperatureB=25 degC  temperatureB_nominal_specify=off  temperatureB_nominal_unit=degC  temperatureB_nominal_value=1  temperatureR_specify=off  temperatureR_priority=High  temperatureR=25 degC  temperatureR_nominal_specify=off  temperatureR_nominal_unit=degC  temperatureR_nominal_value=1
      settings: SourceProductBaseCode=PS  InternalSimscapePortConfiguration="{\"Bottom\":[],\"Left\":[{\"id\":\"a1\",\"label\":\"a1\",\"type\":\"foundation.electrical.electrical\"},{\"id\":\"a2\",\"label\":\"a2\",\"type\":\"foundation.electrical.electrical\"},{\"id\":\"b1\",\"label\":\"b1\",\"type\":\"foundation.electrical.electrical\"},{\"id\":\"b2\",\"label\":\"b2\",\"type\":\"foundation.electrical.electrical\"}],\"Right\":[{\"id\":\"pu_output\",\"label\":\"pu\",\"type\":\"output\"},{\"id\":\"R\",\"label\":\"R\",\"type\":\"foundation.mechanical.rotational.rotational\"},{\"id\":\"C\",\"label\":\"C\",\"type\":\"foundation.mechanical.rotational.rotational\"}],\"Top\":[]}"
  Solver Configuration1 : nesl_utility/Solver Configuration  Commented=on  PhysicalDomain=network_engine_domain  SubClassName=solver  LeftPortType=input  RightPortType=generic  Tones=[]  Harmonics=[]  SimulateNoise=off  Profile=off  UseLocalSampling=off  EnableSwitchedLinearOptims=on  FrequencyDomain=off  UseCCode=off  RelTol=0.001  AbsTol=1e-06  MinStep=1e-09  ToWorkspace=off  RevertToSquareIcSolve=off  NumHomotopyIterations=100  PhasorMode=off  PhasorModeNumHarmonics=1  IndexReductionMethod=DerivativeReplacement  DoDC=off  ResidualTolerance=1e-9  UseLocalSolver=on  LocalSolverChoice=NE_BACKWARD_EULER_ADVANCER  LocalSolverSampleTime=Ts  DoFixedCost=on  MaxNonlinIter=4  MaxModeIter=2  ComputeImpulses=off  ImpulseIterations=2  LinearAlgebra=auto  LinearAlgebraNumThread=0  EquationFormulation=NE_TIME_EF  DelaysMemoryBudget=1024  AutomaticFiltering=on  FilteringTimeConstant=0.001  PartitionStorageMethod=AS_NEEDED  PartitionMemoryBudget=1024  PartitionMethod=FAST
      settings: SourceProductBaseCode=SS,PW,VE
  Solver Configuration4 : nesl_utility/Solver Configuration  Commented=on  PhysicalDomain=network_engine_domain  SubClassName=solver  LeftPortType=input  RightPortType=generic  Tones=[]  Harmonics=[]  SimulateNoise=off  Profile=off  UseLocalSampling=off  EnableSwitchedLinearOptims=on  FrequencyDomain=off  UseCCode=off  RelTol=0.001  AbsTol=1e-06  MinStep=1e-09  ToWorkspace=off  RevertToSquareIcSolve=off  NumHomotopyIterations=100  PhasorMode=off  PhasorModeNumHarmonics=1  IndexReductionMethod=DerivativeReplacement  DoDC=off  ResidualTolerance=1e-9  UseLocalSolver=on  LocalSolverChoice=NE_BACKWARD_EULER_ADVANCER  LocalSolverSampleTime=Ts/cnt_pTs  DoFixedCost=on  MaxNonlinIter=4  MaxModeIter=2  ComputeImpulses=off  ImpulseIterations=2  LinearAlgebra=auto  LinearAlgebraNumThread=0  EquationFormulation=NE_TIME_EF  DelaysMemoryBudget=1024  AutomaticFiltering=on  FilteringTimeConstant=0.001  PartitionStorageMethod=AS_NEEDED  PartitionMemoryBudget=1024  PartitionMethod=FAST
      settings: SourceProductBaseCode=SS,PW,VE
  Solver Configuration5 : nesl_utility/Solver Configuration  Commented=on  PhysicalDomain=network_engine_domain  SubClassName=solver  LeftPortType=input  RightPortType=generic  Tones=[]  Harmonics=[]  SimulateNoise=off  Profile=off  UseLocalSampling=off  EnableSwitchedLinearOptims=on  FrequencyDomain=off  UseCCode=off  RelTol=0.001  AbsTol=1e-06  MinStep=1e-09  ToWorkspace=off  RevertToSquareIcSolve=off  NumHomotopyIterations=100  PhasorMode=off  PhasorModeNumHarmonics=1  IndexReductionMethod=DerivativeReplacement  DoDC=off  ResidualTolerance=1e-9  UseLocalSolver=on  LocalSolverChoice=NE_BACKWARD_EULER_ADVANCER  LocalSolverSampleTime=Ts/cnt_pTs  DoFixedCost=on  MaxNonlinIter=4  MaxModeIter=2  ComputeImpulses=off  ImpulseIterations=2  LinearAlgebra=auto  LinearAlgebraNumThread=0  EquationFormulation=NE_TIME_EF  DelaysMemoryBudget=1024  AutomaticFiltering=on  FilteringTimeConstant=0.001  PartitionStorageMethod=AS_NEEDED  PartitionMemoryBudget=1024  PartitionMethod=FAST
      settings: SourceProductBaseCode=SS,PW,VE
  Step : Step  Commented=on  Time=0.3  After=0.1  SampleTime=0
  Subsystem : Subsystem  Commented=on
      settings: PortSchema="{\"entries\":[{\"content\":{\"sides\":[{\"content\":{\"connectorIds\":[\"In1\",\"In2\",\"In3\"]},\"type\":\"ConnectorPlacement.EquallySpacedRectSide\",\"uuid\":\"ae018a65-5a33-4915-a156-b0f5ff0744c4\"},{\"content\":{\"connectorIds\":[\"RConn1\",\"RConn2\",\"RConn3\"],\"side\":\"RIGHT\"},\"type\":\"ConnectorPlacement.EquallySpacedRectSide\",\"uuid\":\"85679cce-0873-4dc4-89bb-01646651c655\"},{\"content\":{\"connectorIds\":[\"LConn1\"],\"side\":\"TOP\"},\"type\":\"ConnectorPlacement.EquallySpacedRectSide\",\"uuid\":\"b63fd400-b4fa-48a8-be44-71d7511bfdeb\"},{\"content\":{\"connectorIds\":[\"RConn4\"],\"side\":\"BOTTOM\"},\"type\":\"ConnectorPlacement.EquallySpacedRectSide\",\"uuid\":\"d541e435-ee8d-46cd-862f-23d3a68c6ee7\"}]},\"type\":\"ConnectorPlacement.EquallySpacedConnector\",\"uuid\":\"0dd110c0-59c4-48c2-b21b-e2e58ba4e561\"}],\"packageUris\":[\"http://schema.mathworks.com/mf0/Connector/R2020b\"],\"version\":\"1.0\"}"
  Subsystem1 : Subsystem  Commented=on
      settings: PortSchema="{\"entries\":[{\"content\":{\"sides\":[{\"content\":{\"connectorIds\":[\"LConn1\",\"LConn2\",\"LConn3\"]},\"type\":\"ConnectorPlacement.EquallySpacedRectSide\",\"uuid\":\"dbbc7ef1-15e1-407a-bb12-b123d1fc9109\"},{\"content\":{\"connectorIds\":[\"RConn1\",\"RConn2\",\"RConn3\"],\"side\":\"RIGHT\"},\"type\":\"ConnectorPlacement.EquallySpacedRectSide\",\"uuid\":\"8b21e888-66b1-4e2a-b4f7-566dd74beec7\"},{\"content\":{\"connectorIds\":[\"Out1\"],\"side\":\"TOP\"},\"type\":\"ConnectorPlacement.EquallySpacedRectSide\",\"uuid\":\"146dc571-d6b7-44ef-884f-58c1df98455b\"}]},\"type\":\"ConnectorPlacement.EquallySpacedConnector\",\"uuid\":\"d5b044f9-fc85-4040-aea4-b4ba2cc55902\"}],\"packageUris\":[\"http://schema.mathworks.com/mf0/Connector/R2020b\"],\"version\":\"1.0\"}"
  Subsystem10 : Subsystem  Commented=on
      settings: PortSchema="{\"entries\":[{\"content\":{\"sides\":[{\"content\":{\"connectorIds\":[\"LConn1\",\"LConn2\"]},\"type\":\"ConnectorPlacement.EquallySpacedRectSide\",\"uuid\":\"dffb654e-a19d-418f-9ad8-06d1e7de3d45\"},{\"content\":{\"connectorIds\":[\"Out1\"],\"side\":\"RIGHT\"},\"type\":\"ConnectorPlacement.EquallySpacedRectSide\",\"uuid\":\"3b6ff8f3-a1b5-4715-8b2e-8ea31748caf5\"},{\"content\":{\"connectorIds\":[\"LConn3\",\"LConn4\"],\"side\":\"TOP\"},\"type\":\"ConnectorPlacement.EquallySpacedRectSide\",\"uuid\":\"86e0401e-dbf4-4d85-b6ad-4c57f4104f30\"}]},\"type\":\"ConnectorPlacement.EquallySpacedConnector\",\"uuid\":\"e2ddf03f-556d-4982-bd4f-671a8a0b5eb5\"}],\"packageUris\":[\"http://schema.mathworks.com/mf0/Connector/R2020b\"],\"version\":\"1.0\"}"
  Subsystem11 : Subsystem  Commented=on
  Subsystem12 : Subsystem  Commented=on
      settings: PortSchema="{\"entries\":[{\"content\":{\"sides\":[{\"content\":{\"connectorIds\":[\"In1\",\"In2\",\"In3\"]},\"type\":\"ConnectorPlacement.EquallySpacedRectSide\",\"uuid\":\"ae018a65-5a33-4915-a156-b0f5ff0744c4\"},{\"content\":{\"connectorIds\":[\"RConn1\",\"RConn2\",\"RConn3\"],\"side\":\"RIGHT\"},\"type\":\"ConnectorPlacement.EquallySpacedRectSide\",\"uuid\":\"85679cce-0873-4dc4-89bb-01646651c655\"},{\"content\":{\"connectorIds\":[\"LConn1\"],\"side\":\"TOP\"},\"type\":\"ConnectorPlacement.EquallySpacedRectSide\",\"uuid\":\"b63fd400-b4fa-48a8-be44-71d7511bfdeb\"},{\"content\":{\"connectorIds\":[\"RConn4\"],\"side\":\"BOTTOM\"},\"type\":\"ConnectorPlacement.EquallySpacedRectSide\",\"uuid\":\"d541e435-ee8d-46cd-862f-23d3a68c6ee7\"}]},\"type\":\"ConnectorPlacement.EquallySpacedConnector\",\"uuid\":\"0dd110c0-59c4-48c2-b21b-e2e58ba4e561\"}],\"packageUris\":[\"http://schema.mathworks.com/mf0/Connector/R2020b\"],\"version\":\"1.0\"}"
  Subsystem13 : Subsystem
  Subsystem14 : Subsystem
  Subsystem2 : Subsystem  Commented=on
      settings: PortSchema="{\"entries\":[{\"content\":{\"sides\":[{\"content\":{\"connectorIds\":[\"LConn1\",\"LConn2\"]},\"type\":\"ConnectorPlacement.EquallySpacedRectSide\",\"uuid\":\"dffb654e-a19d-418f-9ad8-06d1e7de3d45\"},{\"content\":{\"connectorIds\":[\"Out1\"],\"side\":\"RIGHT\"},\"type\":\"ConnectorPlacement.EquallySpacedRectSide\",\"uuid\":\"3b6ff8f3-a1b5-4715-8b2e-8ea31748caf5\"},{\"content\":{\"connectorIds\":[\"LConn3\",\"LConn4\"],\"side\":\"TOP\"},\"type\":\"ConnectorPlacement.EquallySpacedRectSide\",\"uuid\":\"86e0401e-dbf4-4d85-b6ad-4c57f4104f30\"}]},\"type\":\"ConnectorPlacement.EquallySpacedConnector\",\"uuid\":\"e2ddf03f-556d-4982-bd4f-671a8a0b5eb5\"}],\"packageUris\":[\"http://schema.mathworks.com/mf0/Connector/R2020b\"],\"version\":\"1.0\"}"
  Subsystem3 : Subsystem  Commented=on
  Subsystem4 : Subsystem  Commented=on
      settings: PortSchema="{\"entries\":[{\"content\":{\"sides\":[{\"content\":{\"connectorIds\":[\"In1\",\"In2\",\"In3\"]},\"type\":\"ConnectorPlacement.EquallySpacedRectSide\",\"uuid\":\"ae018a65-5a33-4915-a156-b0f5ff0744c4\"},{\"content\":{\"connectorIds\":[\"RConn1\",\"RConn2\",\"RConn3\"],\"side\":\"RIGHT\"},\"type\":\"ConnectorPlacement.EquallySpacedRectSide\",\"uuid\":\"85679cce-0873-4dc4-89bb-01646651c655\"},{\"content\":{\"connectorIds\":[\"LConn1\"],\"side\":\"TOP\"},\"type\":\"ConnectorPlacement.EquallySpacedRectSide\",\"uuid\":\"b63fd400-b4fa-48a8-be44-71d7511bfdeb\"},{\"content\":{\"connectorIds\":[\"RConn4\"],\"side\":\"BOTTOM\"},\"type\":\"ConnectorPlacement.EquallySpacedRectSide\",\"uuid\":\"d541e435-ee8d-46cd-862f-23d3a68c6ee7\"}]},\"type\":\"ConnectorPlacement.EquallySpacedConnector\",\"uuid\":\"0dd110c0-59c4-48c2-b21b-e2e58ba4e561\"}],\"packageUris\":[\"http://schema.mathworks.com/mf0/Connector/R2020b\"],\"version\":\"1.0\"}"
  Subsystem5 : Subsystem  Commented=on
      settings: PortSchema="{\"entries\":[{\"content\":{\"sides\":[{\"content\":{\"connectorIds\":[\"LConn1\",\"LConn2\",\"LConn3\"]},\"type\":\"ConnectorPlacement.EquallySpacedRectSide\",\"uuid\":\"dbbc7ef1-15e1-407a-bb12-b123d1fc9109\"},{\"content\":{\"connectorIds\":[\"RConn1\",\"RConn2\",\"RConn3\"],\"side\":\"RIGHT\"},\"type\":\"ConnectorPlacement.EquallySpacedRectSide\",\"uuid\":\"8b21e888-66b1-4e2a-b4f7-566dd74beec7\"},{\"content\":{\"connectorIds\":[\"Out1\"],\"side\":\"TOP\"},\"type\":\"ConnectorPlacement.EquallySpacedRectSide\",\"uuid\":\"146dc571-d6b7-44ef-884f-58c1df98455b\"}]},\"type\":\"ConnectorPlacement.EquallySpacedConnector\",\"uuid\":\"d5b044f9-fc85-4040-aea4-b4ba2cc55902\"}],\"packageUris\":[\"http://schema.mathworks.com/mf0/Connector/R2020b\"],\"version\":\"1.0\"}"
  Subsystem6 : Subsystem  Commented=on
  Subsystem7 : Subsystem  Commented=on
  Subsystem8 : Subsystem  Commented=on
      settings: PortSchema="{\"entries\":[{\"content\":{\"sides\":[{\"content\":{\"connectorIds\":[\"LConn1\",\"LConn2\",\"LConn3\"]},\"type\":\"ConnectorPlacement.EquallySpacedRectSide\",\"uuid\":\"dffb654e-a19d-418f-9ad8-06d1e7de3d45\"},{\"content\":{\"connectorIds\":[\"Out1\"],\"side\":\"RIGHT\"},\"type\":\"ConnectorPlacement.EquallySpacedRectSide\",\"uuid\":\"3b6ff8f3-a1b5-4715-8b2e-8ea31748caf5\"},{\"content\":{\"connectorIds\":[\"LConn4\"],\"side\":\"TOP\"},\"type\":\"ConnectorPlacement.EquallySpacedRectSide\",\"uuid\":\"86e0401e-dbf4-4d85-b6ad-4c57f4104f30\"}]},\"type\":\"ConnectorPlacement.EquallySpacedConnector\",\"uuid\":\"e2ddf03f-556d-4982-bd4f-671a8a0b5eb5\"}],\"packageUris\":[\"http://schema.mathworks.com/mf0/Connector/R2020b\"],\"version\":\"1.0\"}"
  Subsystem9 : Subsystem  Commented=on
  Sum : Sum  Commented=on  Inputs=|+-
  Sum1 : Sum  Commented=on  Inputs=|+-
  Sum2 : Sum  Commented=on  Inputs=|+-
  Surface Mount PMSM : autolibpmsmexterior/Surface Mount PMSM  Commented=on  port_config=Torque  sim_type=Discrete  Ts=Ts  FilePath=E:\Sandbox\Bauto\Work\surfacepmsm_motordata.m  P=P  Rs=Rs  Ldq_=Ls  KConstText=Permanent flux linkage constant (lambda_pm):  lambda_pm=Flux  Ke=159.9771  Kt=1.323  mechanical=[0.00001, 4.924e-5, 0]  idq0=[0 0]  theta_init=0  omega_init=0  KConst=Flux  lambda_pm_calc=Flux  RefBlkName='autolibpmsmexterior/Surface Mount PMSM'  aMode=1  Ldq="[0.0003752   0.0003752]"
      settings: SourceProductBaseCode=PW,DR,MT,VE
  Theta : Goto  Commented=on  GotoTag=Theta
  Three-Phase Inverter1 : Subsystem  Commented=on
  Tload1 : Subsystem  Commented=on
  Tload3 : Subsystem  Commented=on
  Torque Source1 : fl_lib/Mechanical/Mechanical Sources/Ideal Torque Source  Commented=on
      settings: SourceProductBaseCode=PW,SS,VE
  Torque Source3 : fl_lib/Mechanical/Mechanical Sources/Ideal Torque Source  Commented=on
      settings: SourceProductBaseCode=PW,SS,VE
  TxTy : MATLAB Function  TreatAsAtomicUnit=on
  TxTy1 : MATLAB Function  TreatAsAtomicUnit=on
  Unit Delay : UnitDelay  Commented=on  SampleTime=Ts  HasFrameUpgradeWarning=on
  XYZ : MATLAB Function  TreatAsAtomicUnit=on
  a : Constant  Commented=on  Value=0.5
  a1 : Constant  Commented=on  Value=0.5
  b : Constant  Commented=on  Value=0.5
  clark : Subsystem  Commented=on
  ref_ratio : Subsystem  Commented=on
  wires:
  Inverse_Park/1(Vα) -> Goto3/1, SVPWM/1(Vα)
  Inverse_Park/2(Vβ) -> Goto4/1, SVPWM/2(Vβ)
  Constant3/1 -> SVPWM/3(Vbus)
  Constant2/1 -> SVPWM/4(TS)
  Constant4/1 -> Average-Value Inverter/2
  Step/1 -> Surface Mount PMSM/1
  Mux/1 -> Duty_conver/1(In1)
  SVPWM/1(Ta) -> Mux/1, Scope3/1
  SVPWM/2(Tb) -> Mux/2, Scope3/2
  SVPWM/3(Tc) -> Scope3/3, Mux/3
  Duty_conver/1(Out1) -> Average-Value Inverter/1, Gain2/1, Scope6/1
  Surface Mount PMSM/1 -> Bus Selector/1
  Bus Selector/1 -> Gain/1  "<MtrSpd>"
  Bus Selector/2 -> Gain1/1, Scope7/1  "<MtrPos>"
  Bus Selector/3 -> Scope8/1  "<MtrTrq>"
  Gain/1 -> Goto2/1, Scope9/1
  Gain1/1 -> Mod/1
  Mod/1 -> Scope7/2, Theta/1
  Constant6/1 -> Mod/2
  Surface Mount PMSM/2 -> Demux1/1, Crrent/1
  From1/1 -> clark/1(PhI)
  clark/1(Iα) -> Scope/1, Goto5/1, Park/1(Iα)
  clark/2(Iβ) -> Scope/2, Goto6/1, Park/2(Iβ)
  From2/1 -> SinCos1/1
  SinCos1/1 -> Park/3(Sin_Theta)
  SinCos1/2 -> Park/4(Cos_Theta)
  Park/1(Id) -> Goto/1
  Park/2(Iq) -> Goto1/1
  Bus Selector/4 -> Scope2/1, Scope1/1  "<IdSync>"
  Bus Selector/5 -> Scope11/1, Scope2/2  "<IqSync>"
  Sum/1 -> PID Controller/1
  From3/1 -> Sum/2
  From4/1 -> Sum1/2
  Constant7/1 -> Sum/1
  PID Controller2/1 -> Scope12/3, Inverse_Park/2(Vq)
  Sum1/1 -> PID Controller2/1
  PID Controller/1 -> Scope12/2, Inverse_Park/1(Vd)
  PID Controller1/1 -> Scope12/1, Sum1/1
  Sum2/1 -> Scope12/4, PID Controller1/1
  From5/1 -> Sum2/2
  Signal Builder/1(Signal 1) -> Gain3/1
  ? -> ?
  Gain2/1 -> Surface Mount PMSM/2
  From6/1 -> SMO/1(Valpha)
  From7/1 -> SMO/2(Vbeta)
  From8/1 -> SMO/3(Ialpha)
  From9/1 -> SMO/4(Ibeta)
  From10/1 -> SMO/5(theta)
  From12/1 -> SMO/6(V)
  Constant8/1 -> SVPWM1/3(Vbus)
  Constant9/1 -> SVPWM1/4(TS)
  SVPWM1/1(Ta) -> Mux1/1, Scope4/1
  SVPWM1/2(Tb) -> Mux1/2, Scope4/2
  SVPWM1/3(Tc) -> Mux1/3, Scope4/3
  Mux1/1 -> Duty_conver1/1(In1)
  Duty_conver1/1(Out1) -> Scope5/1
  Demux1/3 -> Scope10/2
  Bus Selector/8 -> Scope10/1  "<IcStator>"
  From13/1 -> Scope1/2
  From15/1 -> Scope11/2
  Constant1/1 -> Sum2/1
  2Phase_D1D2/1(D1) -> 2Phase_T/2(D1), Mux3/2
  2Phase_D1D2/2(D2) -> Scope16/1, Mux3/1, 2Phase_T/3(D2)
  Sector1/1(N) -> Scope16/3, Scope14/3, Scope17/4, Scope13/3, 2Phase_T/1(N), 2Phase_D1D2/3(N)
  Mux2/1 -> Scope27/1, Average-Value Inverter1/1, Scope14/1, Scope19/1
  Mux3/1 -> Scope15/1, Scope14/2
  PWM_Generator/1(pwm1) -> Scope17/1, Subsystem/1(pwm1)
  PWM_Generator/2(pwm2) -> Scope17/2, Subsystem/2(pwm2)
  PWM_Generator/3(pwm3) -> Scope17/3, Subsystem/3(pwm3)
  Constant10/1 -> Average-Value Inverter1/2
  Average-Value Inverter1/1 -> Demux/1
  Subsystem1/1(Out1) -> Demux2/1, Scope20/1
  Subsystem6/1(OUT) -> Scope25/1
  Subsystem7/1(OUT) -> Scope26/1
  From18/1 -> Scope24/2
  From17/1 -> Scope24/1
  Sensing trq1/1(Tq) -> Goto10/1
  Sensing trq1/2(w) -> Goto9/1
  Subsystem5/1(Out1) -> Scope18/1
  Subsystem2/1(OUT) -> Scope22/1
  Demux/1 -> Add4/1, Scope21/1
  Demux/2 -> Add5/1, Scope21/2
  Demux/3 -> Add4/2, Add5/2, Scope21/3
  Subsystem3/1(OUT) -> Scope23/1
  2Phase_T/1(Da) -> Scope28/2, Da-Dc/1, PWM_Generator/1(D1), Mux2/1
  2Phase_T/2(Db) -> Scope28/3, Db-Dc/1, PWM_Generator/2(D2), Mux2/2
  2Phase_T/3(Dc) -> Scope28/4, Db-Dc/2, Da-Dc/2, PWM_Generator/3(D3), Mux2/3
  Unit Delay/1 -> 2Phase_D1D2/1(alpha), Scope13/2, Sector1/1(Alpha), Scope16/2, ref_ratio/1(alpha)
  Demux2/3 -> Add2/2, Add3/2
  Demux2/2 -> Add6/2, Add3/1
  Demux2/1 -> Add6/1, Add2/1
  Add2/1 -> Scope29/1
  Add3/1 -> Scope29/2
  Subsystem8/1(OUT) -> Scope30/1
  Db-Dc/1 -> Scope19/3
  Da-Dc/1 -> Scope19/2
  Add4/1 -> Scope31/1
  Add5/1 -> Scope31/2
  Subsystem9/1(OUT) -> Scope32/1
  Subsystem11/1(OUT) -> Scope34/1
  Subsystem10/1(OUT) -> Scope33/1
  Add6/1 -> Scope29/3
  From14/1 -> Scope35/1
  From16/1 -> Scope35/2
  Sensing trq3/2(w) -> Goto8/1
  Sensing trq3/1(Tq) -> Goto7/1
  a/1 -> ref_ratio/2(lead)
  b/1 -> ref_ratio/3(leg)
  a1/1 -> 2Phase_D1D2/2(m)
  Repeating Sequence1/1 -> Unit Delay/1
  From19/1 -> Scope36/1
  Gain4/1 -> PWM_Generator1/3(D3)
  Gain5/1 -> PWM_Generator1/2(D2)
  Gain6/1 -> PWM_Generator1/1(D1)
  XYZ/1(X) -> Scope41/1, TxTy/2(X)
  XYZ/2(Y) -> Scope41/2, TxTy/3(Y)
  XYZ/3(Z) -> Scope41/3, TxTy/4(Z)
  SinCos/2 -> Inverse_Park1/4(cos_theta)
  SinCos/1 -> Inverse_Park1/3(sin_theta)
  D/1 -> Inverse_Park1/1(Vd)
  Q/1 -> Inverse_Park1/2(Vq)
  Q1/1 -> XYZ/3(Ud)
  Inverse_Park1/1(Vα) -> Sector2/1(Vα), Sector/1(Ualpha), XYZ/1(Ualpha)
  Inverse_Park1/2(Vβ) -> Sector2/2(Vβ), Sector/2(Ubeta), XYZ/2(Ubeta)
  Q2/1 -> XYZ/4(Ts)
  Q3/1 -> TxTy/5(Ts)
  TxTy/1(Tx) -> TxTy1/2(T1), Scope38/1
  TxTy/2(Ty) -> TxTy1/3(T2), Scope38/2
  SinCos2/1 -> Inverse_Park/3(sin_theta)
  From20/1 -> SinCos2/1
  SinCos2/2 -> Inverse_Park/4(cos_theta)
  Q4/1 -> TxTy1/5(Ts)
  TxTy/3(T0) -> TxTy1/4(T0)
  TxTy1/2(Tb) -> Subsystem14/2(B), Scope39/2
  TxTy1/1(Ta) -> Subsystem14/1(A), Scope39/1
  TxTy1/3(Tc) -> Subsystem14/3(C), Scope39/3
  Sector2/1(N) -> Scope40/3
  Sector/1(y) -> Scope44/3, Scope39/4, TxTy1/1(N), TxTy/1(N)
  Repeating Sequence3/1 -> Subsystem14/4(Theta), SinCos/1
  Subsystem14/1(D) -> Scope45/2  "D"
  Subsystem14/2(Q) -> Scope45/3  "Q"
  SinCos3/2 -> Sector3/5(costheta)
  Repeating Sequence4/1 -> Subsystem13/4(Theta), SinCos3/1
  SinCos3/1 -> Sector3/4(sintheta)
  Constant/1 -> Sector3/3(Ud)
  Constant11/1 -> Sector3/2(Vq)
  Constant5/1 -> Sector3/1(Vd)
  Subsystem13/1(D) -> Scope37/2  "D"
  Subsystem13/2(Q) -> Scope37/3  "Q"
  Sector3/1(Ta) -> Subsystem13/1(A)
  Sector3/2(Tb) -> Subsystem13/2(B)
  Sector3/3(Tc) -> Subsystem13/3(C)
  connections:
  Electrical Reference1/LConn1 -- DC Voltage Source/RConn1
  DC Voltage Source/LConn1 -- Subsystem/LConn1
  Subsystem/RConn4 -- Electrical Reference/LConn1
  Subsystem1/LConn1 -- Subsystem8/LConn1 -- Subsystem3/LConn1 -- Subsystem/RConn1
  Subsystem1/LConn2 -- Subsystem8/LConn2 -- Subsystem3/LConn2 -- Subsystem/RConn2
  Subsystem1/LConn3 -- Subsystem8/LConn3 -- Subsystem3/LConn3 -- Subsystem/RConn3 -- Subsystem8/LConn4
  Electrical Reference3/LConn1 -- Subsystem3/LConn4
  Inertia1/LConn1 -- Torque Source1/LConn1 -- Sensing trq1/RConn1
  "Single-Phase Asynchronous Machine (fundamental, SI)1"/LConn3 -- Subsystem5/RConn3 -- Subsystem6/LConn3
  Solver Configuration1/RConn1 -- MRRef Load1/LConn1 -- Torque Source1/RConn2
  "Single-Phase Asynchronous Machine (fundamental, SI)1"/LConn2 -- "Single-Phase Asynchronous Machine (fundamental, SI)1"/LConn4 -- Subsystem5/RConn2 -- Subsystem6/LConn2
  Subsystem4/RConn2 -- Subsystem5/LConn2 -- Subsystem7/LConn2
  Subsystem4/RConn3 -- Subsystem5/LConn3 -- Subsystem7/LConn3
  Subsystem4/RConn1 -- Subsystem5/LConn1 -- Subsystem7/LConn1
  "Single-Phase Asynchronous Machine (fundamental, SI)1"/LConn1 -- Subsystem5/RConn1 -- Subsystem6/LConn1
  Electrical Reference6/LConn1 -- Subsystem7/LConn4
  MRRef IPMSM1/LConn1 -- "Single-Phase Asynchronous Machine (fundamental, SI)1"/RConn3
  Electrical Reference4/LConn1 -- Subsystem4/RConn4
  Tload1/RConn1 -- Torque Source1/RConn1
  DC Voltage Source1/LConn1 -- Subsystem4/LConn1
  Electrical Reference5/LConn1 -- Subsystem6/LConn4
  Sensing trq1/LConn1 -- "Single-Phase Asynchronous Machine (fundamental, SI)1"/RConn2
  Subsystem2/LConn2 -- Inductor3/LConn1 -- Subsystem1/RConn3 -- Subsystem9/LConn2
  Subsystem1/RConn1 -- Subsystem9/LConn1 -- Inductor4/LConn1 -- Subsystem2/LConn1
  Electrical Reference7/LConn1 -- Subsystem9/LConn4
  Resistor2/LConn1 -- Subsystem11/LConn2 -- Inductor3/RConn1 -- Subsystem10/LConn2
  Resistor3/LConn1 -- Subsystem11/LConn1 -- Inductor4/RConn1 -- Subsystem10/LConn1
  Electrical Reference8/LConn1 -- Subsystem11/LConn4
  Resistor2/RConn1 -- Subsystem2/LConn3 -- Subsystem2/LConn4 -- Subsystem1/RConn2 -- Subsystem9/LConn3 -- Subsystem11/LConn3 -- Subsystem10/LConn4 -- Subsystem10/LConn3 -- Solver Configuration4/RConn1 -- Resistor3/RConn1
  Torque Source3/LConn1 -- Inertia3/LConn1 -- Sensing trq3/RConn1
  MRRef Load3/LConn1 -- Solver Configuration5/RConn1 -- Torque Source3/RConn2
  "Single-Phase Asynchronous Machine (fundamental, SI)4"/LConn2 -- "Single-Phase Asynchronous Machine (fundamental, SI)4"/LConn4
  Tload3/RConn1 -- Torque Source3/RConn1
  "Single-Phase Asynchronous Machine (fundamental, SI)4"/RConn3 -- MRRef IPMSM3/LConn1
  "Single-Phase Asynchronous Machine (fundamental, SI)4"/RConn2 -- Sensing trq3/LConn1
